simulink model "mock_pedestrian_detection_system_2017a"  (R2017a)
settings: Solver=VariableStepAuto  StartTime=0.0  StopTime=100  RelTol=1e-3
libraries: simulink x16, ProSivic_Sensors x9, ProSivic_Commands x3, simulink_extras x1, realtime_pacer_lib x1
settings Model: Creator=Markus Borg  LastModifiedBy=Markus Borg
settings DataIOCC: ReturnWorkspaceOutputs=on
settings SFSimCC: SimUseLocalCustomCode=on
settings RTWCC: RTWUseLocalCustomCode=on

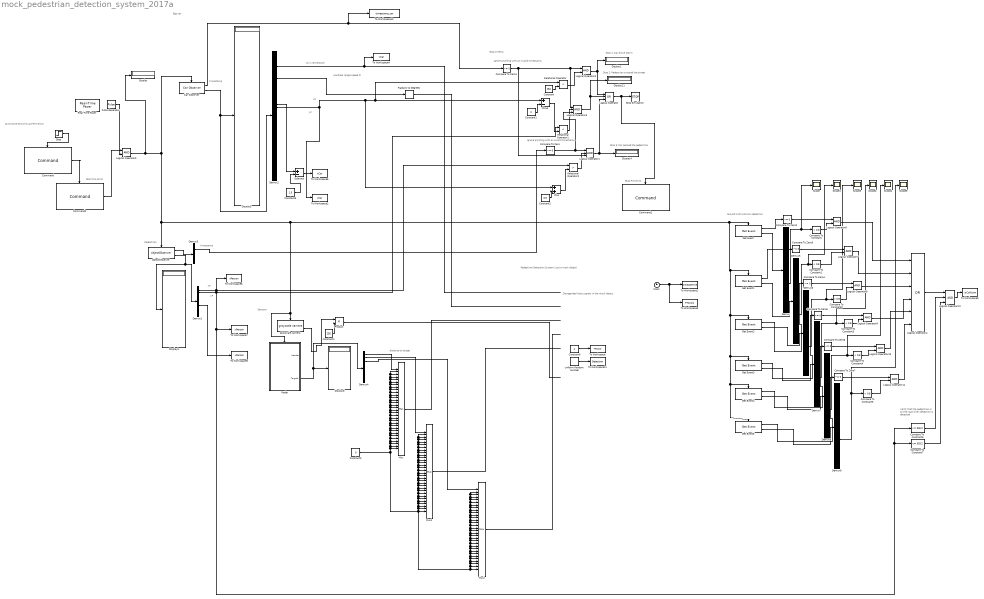
== system mock_pedestrian_detection_system_2017a ==
  note: Disregarded input signals in the mock object
  note: Ground truth collision detection
  note: Syncronize Simulink and Pro-SiVIC
  note: Stop criteria
  note: yP
  note: yC
  note: xP
  note: xC
  note: Ego car
  note: Sensors
  note: Pedestrian
  note: yawRate (angle speed Z)
  note: timestamp
  note: Ignore anything with an invalid timestamp
  note: Pedestrian Detection System (just a mock object)
  note: vC (x dimension)
  note: distance to target
  note: timestamp
  note: Ignore anything with an invalid timestamp
  note: Stop 1: Car drove 100 m
  note: Stop 2: Pedestrian crossed the street
  note: Stop 3: Car passed the pedestrian
  note: Stop Pro-SiVIC
  note: Start Pro-SiVIC
  note: Verify that the pedestrian is on the road when detection is detected
  " grayscale camera" : ProSivic_Sensors/ grayscale camera  topic=dashcam/cam  h=375  w=500  color=on
  Car Observer : ProSivic_Sensors/Car Observer  SystemSampleTime=-1
      link override S-Function: topic=ego_car_obs/car_obs
  Clock : Clock
  Command : ProSivic_Commands/Command  command=SYNCHRODDS  ip=localhost
  Command1 : ProSivic_Commands/Command  command=STOP  ip=localhost
  Command2 : ProSivic_Commands/Command  command=PLAY  ip=localhost
  Compare To Constant{,1..5} (6 alike) : simulink/Logic and Bit Operations/Compare To Constant  relop=<  const=0.8  OutDataTypeStr=boolean
  Compare To Constant6 : simulink/Logic and Bit Operations/Compare To Constant  relop=>=  const=300.2  OutDataTypeStr=boolean
  Compare To Constant7 : simulink/Logic and Bit Operations/Compare To Constant  relop=<=  const=303.2  OutDataTypeStr=boolean
  Compare To Zero{,1..7} (8 alike) : simulink/Logic and Bit Operations/Compare To Zero  relop=~=  OutDataTypeStr=boolean
  Constant : Constant  Value=184
  Constant1 : Constant  Value=2
  Constant2 : Constant  Value=3.6
  Constant3 : Constant  Value=0
  Constant4 : Constant  Value=255
  Constant5 : Constant  Value=1.3
  Constant6 : Constant  Value=4
  Demux{,5..9} (6 alike) : Demux  Outputs=22
  Demux1 : Demux  Outputs=10
  Demux2 : Demux  Outputs=40
  Demux3 : Demux  Outputs=2
  Demux4 : Demux  Outputs=8
  Display{,1,3..6,11} (7 alike) : Display
  Get Event{,1..5} (6 alike) : ProSivic_Sensors/Get Event  eventname=col_event_1
  Logical Operator : Logic  Operator=OR  Inputs=3  AllPortsSameDT=off  OutDataTypeStr=boolean
  Logical Operator1 : Logic  Inputs=3  AllPortsSameDT=off  OutDataTypeStr=boolean
  Logical Operator{2,5..11} (8 alike) : Logic  AllPortsSameDT=off  OutDataTypeStr=boolean
  Logical Operator12 : Logic  Inputs=3  AllPortsSameDT=off  OutDataTypeStr=boolean
  Logical Operator3 : Logic  Inputs=3  AllPortsSameDT=off  OutDataTypeStr=boolean
  Logical Operator4 : Logic  Operator=OR  Inputs=6  AllPortsSameDT=off  OutDataTypeStr=boolean
  Minus : Sum  Inputs=+-
  Mux : Mux  Inputs=32
  Mux1 : Mux  Inputs=32
  Mux2 : Mux  Inputs=32
  Plus : Sum
  Product : Product  OutDataTypeStr=uint8
  Pulse Generator : DiscretePulseGenerator  PulseType=Time based  Period=0.005  PulseWidth=50
  Radar : Subsystem  Description=Radar block retreives the latest radar information from the ProSiVIC DDS store.  AncestorBlock=ProSivic_Sensors/Radar  TreatAsAtomicUnit=on
  Radians to Degrees : simulink_extras/Transformations/Radians to Degrees
  Real-Time Pacer : realtime_pacer_lib/Real-Time Pacer  simTimePerRealTime=10
  Relational Operator : RelationalOperator  Operator=<  OutDataTypeStr=boolean  RndMeth=Simplest
  Relational Operator1 : RelationalOperator  Operator=<  OutDataTypeStr=boolean  RndMeth=Simplest
  Relational Operator2 : RelationalOperator  Operator=>  OutDataTypeStr=boolean  RndMeth=Simplest
  Scope{,1..5} (6 alike) : Scope
  Step : Step  SampleTime=0
  Stop Simulation : Stop
  Subtract : Sum  Inputs=+-
  To Workspace : ToWorkspace  VariableName=TTCcol  SaveFormat=Structure  SampleTime=-1
  To Workspace1 : ToWorkspace  VariableName=SimStopTime  SaveFormat=Structure With Time  SampleTime=-1
  To Workspace10 : ToWorkspace  VariableName=timestamp_car  SaveFormat=Structure With Time  SampleTime=-1
  To Workspace11 : ToWorkspace  VariableName=Detection  SaveFormat=Structure With Time  SampleTime=-1
  To Workspace2 : ToWorkspace  VariableName=yCar  SaveFormat=Structure With Time  SampleTime=-1
  To Workspace3 : ToWorkspace  VariableName=TTCcol1  SaveFormat=Structure  SampleTime=-1
  To Workspace4 : ToWorkspace  VariableName=vCar  SaveFormat=Structure With Time  SampleTime=-1
  To Workspace5 : ToWorkspace  VariableName=xCar  SaveFormat=Structure With Time  SampleTime=-1
  To Workspace6 : ToWorkspace  VariableName=xPerson  SaveFormat=Structure With Time  SampleTime=-1
  To Workspace7 : ToWorkspace  VariableName=yPerson  SaveFormat=Structure With Time  SampleTime=-1
  To Workspace8 : ToWorkspace  VariableName=vPerson  SaveFormat=Structure With Time  SampleTime=-1
  To Workspace9 : ToWorkspace  VariableName=isCollision  SaveFormat=Structure  SampleTime=-1
  Uniform Random Number : UniformRandomNumber  Minimum=0  SampleTime=0.1
  objectObserver : ProSivic_Sensors/objectObserver  topic=ped_obs
  wires:
  Demux1/1 -> To Workspace6/1, Relational Operator2/1
  Constant/1 -> Relational Operator/2
  objectObserver/2 -> Display3/1, Demux1/1
  Constant1/1 -> Minus/2
  Demux1/2 -> Compare To Constant7/1, Compare To Constant6/1, To Workspace7/1, Relational Operator1/1
  Car Observer/2 -> Demux2/1, Display5/1
  Demux2/17 -> To Workspace2/1, Plus/1, Relational Operator/1, Minus/1
  objectObserver/1 -> Demux3/1
  Compare To Zero/1 -> Logical Operator3/3, Logical Operator1/1
  Logical Operator1/1 -> Logical Operator/3, Display4/1
  Clock/1 -> To Workspace3/1, To Workspace1/1
  Constant6/1 -> To Workspace/1
  Demux2/6 -> Radians to Degrees/1
  Radar/2(Target1) -> Demux4/1, Display6/1
  Demux4/1 -> Mux/1
  Mux/1 -> ?
  Demux4/2 -> Mux1/1
  Mux1/1 -> ?
  Mux2/1 -> ?
  Demux4/3 -> Mux2/1
  Constant3/1 -> Mux2/32, Mux2/31, Mux2/30, Mux2/29, Mux2/28, Mux2/27, Mux2/25, Mux2/24, Mux2/23, Mux2/22, Mux2/21, Mux2/20, Mux2/19, Mux2/18, Mux2/17, Mux2/16, Mux2/15, Mux2/14, Mux2/13, Mux2/12, Mux2/11, Mux2/10, Mux2/9, Mux2/8, Mux2/7, Mux2/6, Mux2/5, Mux2/4, Mux2/3, Mux2/2, Mux2/26, Mux1/32, Mux1/31, Mux1/30, Mux1/29, Mux1/28, Mux1/27, Mux1/25, Mux1/24, Mux1/23, Mux1/22, Mux1/21, Mux1/20, Mux1/19, Mux1/18, Mux1/17, Mux1/16, Mux1/15, Mux1/14, Mux1/13, Mux1/12, Mux1/11, Mux1/10, Mux1/9, Mux1/8, Mux1/7, Mux1/6, Mux1/5, Mux1/4, Mux1/3, Mux1/2, Mux1/26, Mux/32, Mux/31, Mux/30, Mux/29, Mux/28, Mux/27, Mux/25, Mux/24, Mux/23, Mux/22, Mux/21, Mux/20, Mux/19, Mux/18, Mux/17, Mux/16, Mux/15, Mux/14, Mux/13, Mux/12, Mux/11, Mux/10, Mux/9, Mux/8, Mux/7, Mux/6, Mux/5, Mux/4, Mux/3, Mux/2, Mux/26
  " grayscale camera"/2 -> Product/1
  Constant4/1 -> Product/2
  Product/1 -> ?
  Radians to Degrees/1 -> ?
  Compare To Zero1/1 -> Logical Operator1/3, Logical Operator3/1, Logical Operator2/1
  Relational Operator/1 -> Logical Operator2/2
  Logical Operator2/1 -> Display1/1, Logical Operator/1
  Car Observer/1 -> To Workspace10/1, Compare To Zero1/1
  Relational Operator1/1 -> Logical Operator3/2
  Logical Operator3/1 -> Display11/1, Logical Operator/2
  Minus/1 -> Relational Operator1/2
  Constant2/1 -> Plus/2
  Relational Operator2/1 -> Logical Operator1/2
  Plus/1 -> Relational Operator2/2
  Demux1/7 -> To Workspace8/1
  Demux3/1 -> Compare To Zero/1
  Command2/1 -> Logical Operator5/1
  Step/1 -> Command/Trigger
  Pulse Generator/1 -> Logical Operator5/2
  Command/1 -> Command2/Trigger
  Logical Operator5/1 -> Display/1, Get Event5/Trigger, Get Event4/Trigger, Get Event3/Trigger, Get Event2/Trigger, Get Event1/Trigger, Get Event/Trigger, Radar/Trigger, " grayscale camera"/Trigger, objectObserver/Trigger, Car Observer/Trigger
  Demux2/1 -> To Workspace4/1
  Logical Operator/1 -> Command1/Trigger, Stop Simulation/1
  Demux/15 -> Scope/1, Compare To Constant/1
  Get Event/2 -> Demux/1
  Demux5/15 -> Scope1/1, Compare To Constant1/1
  Demux6/15 -> Scope3/1, Compare To Constant2/1
  Demux7/15 -> Scope2/1, Compare To Constant3/1
  Demux8/15 -> Scope4/1, Compare To Constant4/1
  Demux9/15 -> Scope5/1, Compare To Constant5/1
  Get Event1/2 -> Demux5/1
  Get Event2/2 -> Demux6/1
  Get Event3/2 -> Demux7/1
  Get Event4/2 -> Demux8/1
  Get Event5/2 -> Demux9/1
  Get Event/1 -> Compare To Zero2/1
  Compare To Zero2/1 -> Logical Operator6/1
  Compare To Constant/1 -> Logical Operator6/2
  Logical Operator6/1 -> Logical Operator4/1
  Get Event1/1 -> Compare To Zero3/1
  Compare To Zero3/1 -> Logical Operator7/1
  Compare To Constant1/1 -> Logical Operator7/2
  Logical Operator7/1 -> Logical Operator4/2
  Compare To Zero4/1 -> Logical Operator8/1
  Compare To Constant2/1 -> Logical Operator8/2
  Logical Operator8/1 -> Logical Operator4/3
  Compare To Zero5/1 -> Logical Operator9/1
  Compare To Constant3/1 -> Logical Operator9/2
  Logical Operator9/1 -> Logical Operator4/4
  Compare To Zero6/1 -> Logical Operator10/1
  Compare To Constant4/1 -> Logical Operator10/2
  Logical Operator10/1 -> Logical Operator4/5
  Compare To Zero7/1 -> Logical Operator11/1
  Compare To Constant5/1 -> Logical Operator11/2
  Logical Operator11/1 -> Logical Operator4/6
  Get Event2/1 -> Compare To Zero4/1
  Get Event3/1 -> Compare To Zero5/1
  Get Event4/1 -> Compare To Zero6/1
  Get Event5/1 -> Compare To Zero7/1
  Logical Operator4/1 -> Logical Operator12/1
  Logical Operator12/1 -> To Workspace9/1
  Compare To Constant6/1 -> Logical Operator12/2
  Compare To Constant7/1 -> Logical Operator12/3
  Constant5/1 -> Subtract/2
  Demux2/16 -> Subtract/1
  Subtract/1 -> To Workspace5/1
  Uniform Random Number/1 -> To Workspace11/1

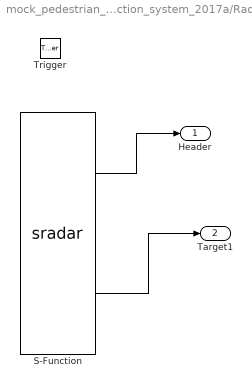
== system mock_pedestrian_detection_system_2017a/Radar ==
  Trigger : TriggerPort  VariantControl=Variant
  S-Function : S-Function  FunctionName=sradar  Parameters=topic,nbmaxtarget  SFunctionDeploymentMode=off  EnableBusSupport=off  mask{topic=radar/radar, nbmaxtarget=1}
      mask prompts: topic "Radar Name"; nbmaxtarget "Number of targets"
  Header : Outport
  Target1 : Outport  Port=2
  wires:
  S-Function/2 -> Target1/1
  S-Function/1 -> Header/1
